simulink model "simulaciont1"  (R2015a)
settings: Solver=ode3  StartTime=0.0  StopTime=10.0  FixedStep=.2  RelTol=1e-3
settings Model: Creator=Jesus  LastModifiedBy=Jesus

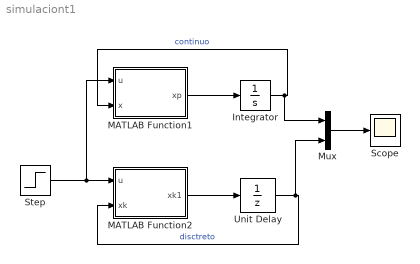
== system simulaciont1 ==
  Integrator : Integrator
  MATLAB Function1 : MATLAB Function  TreatAsAtomicUnit=on
  MATLAB Function2 : MATLAB Function  TreatAsAtomicUnit=on
  Mux : Mux  Inputs=2
  Scope : Scope
  Step : Step  SampleTime=0
  Unit Delay : UnitDelay  SampleTime=-1
  wires:
  Step/1 -> MATLAB Function1/1(u), MATLAB Function2/1(u)
  MATLAB Function1/1(xp) -> Integrator/1
  Integrator/1 -> Mux/1, MATLAB Function1/2(x)  "continuo"
  Unit Delay/1 -> Mux/2, MATLAB Function2/2(xk)  "disctreto"
  MATLAB Function2/1(xk1) -> Unit Delay/1
  Mux/1 -> Scope/1

== matlab function simulaciont1/MATLAB Function1 ==
  data: u input; xp output; x input
function xp = fcn(u,x)
%#codegen

xp=-2*x+2*u;

== matlab function simulaciont1/MATLAB Function2 ==
  data: u input; xk1 output; xk input
function xk1 = fcn(u,xk)
%#codegen

xk1=(0.6703*xk) + (0.3297*u);
